simulink model "Ejemplo_3"  (R2021b)
settings: Solver=VariableStepAuto  StartTime=0.0  StopTime=10.0  RelTol=1e-3
libraries: simulink_extras x3, commrandsrc3 x1
settings Model: Creator=Hagui  LastModifiedBy=Hagui

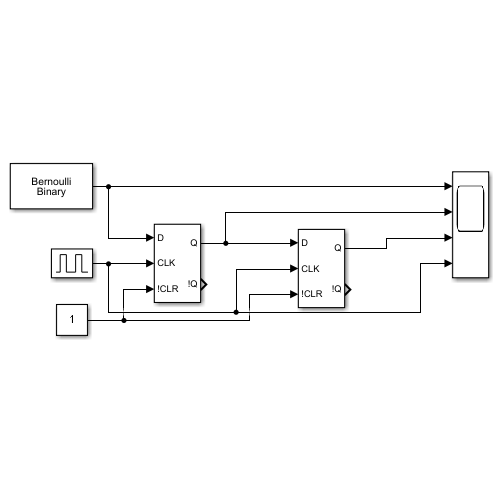
[thumbnail: Simulink's stored preview of the top-level diagram]
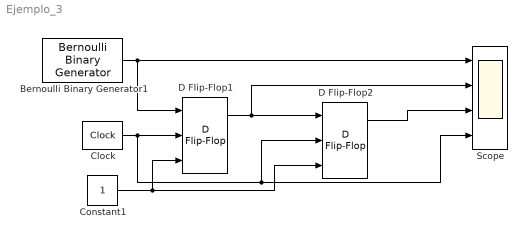
== system Ejemplo_3 ==
  Bernoulli Binary Generator1 : commrandsrc3/Bernoulli Binary Generator  ProbabilityOfZero=0.5  SeedSource=Auto  Seed=0  SampleTime=1  SamplesPerFrame=1  OutputDataType=boolean  SimulateUsing=Interpreted execution
  Clock : simulink_extras/Flip Flops/Clock  period=1
  Constant1 : Constant
  D Flip-Flop1 : simulink_extras/Flip Flops/D Flip-Flop
  D Flip-Flop2 : simulink_extras/Flip Flops/D Flip-Flop
  Scope : Scope  NumInputPorts=4
  wires:
  Constant1/1 -> D Flip-Flop2/3, D Flip-Flop1/3
  Bernoulli Binary Generator1/1 -> D Flip-Flop1/1, Scope/1
  Clock/1 -> D Flip-Flop2/2, Scope/4, D Flip-Flop1/2
  D Flip-Flop2/1 -> Scope/3
  D Flip-Flop1/1 -> D Flip-Flop2/1, Scope/2
